simulink model "final"  (R2024a)
settings: Solver=VariableStepAuto  StartTime=0.0  StopTime=10.0  RelTol=1e-3
values from neighbouring files (symbols this model uses):
  A_air = 0.00588710854841    [run1.mat]    (also in run2.mat)
  Cs = 0.9    [run1.mat]    (also in run2.mat)
  h = 0.0127000254001    [run1.mat]    (also in run2.mat)
  m = 100    [run1.mat]    (also in run2.mat)
  T_f = 21    [run1.mat]    (also in run2.mat)
libraries: slctrl_linear x2, slpidlib x1
settings Model: Creator=veswaranandam  LastModifiedBy=veswaranandam

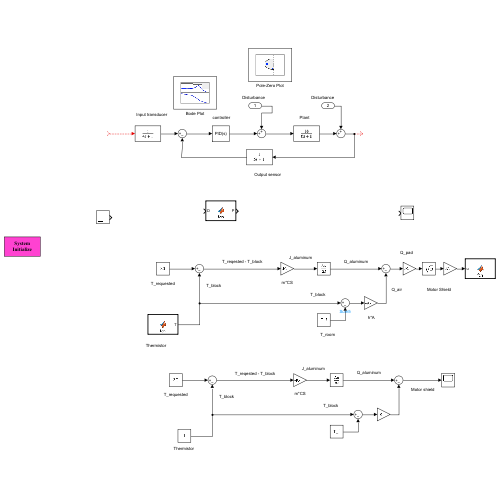
[thumbnail: Simulink's stored preview of the top-level diagram]
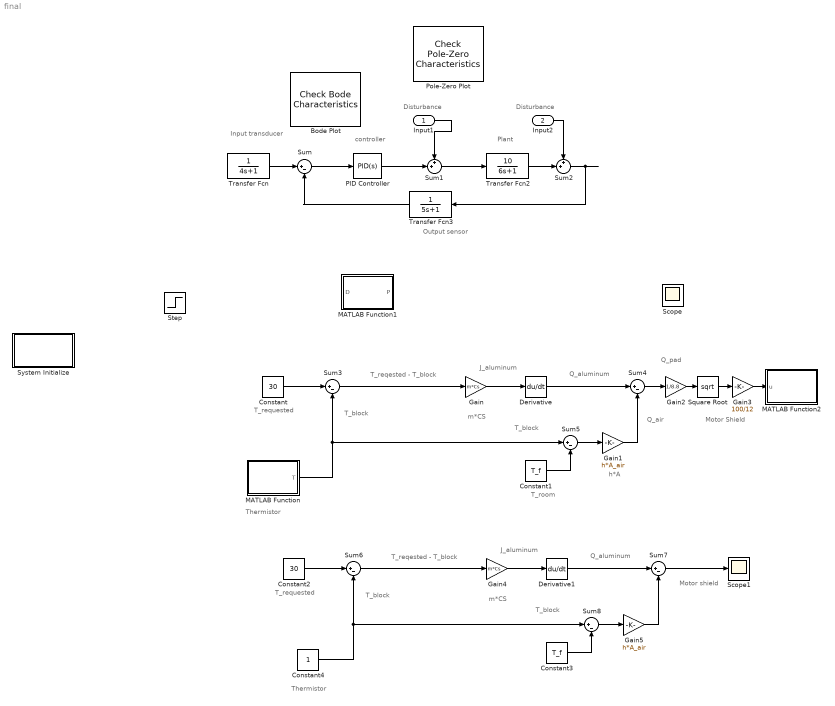
== system final ==
  note: Motor shield
  note: Thermistor
  note: T_block
  note: h*A
  note: T_room
  note: Q_pad
  note: Q_air
  note: Q_aluminum
  note: J_aluminum
  note: m*CS
  note: T_reqested - T_block
  note: T_block
  note: T_requested
  note: Motor Shield
  note: Thermistor
  note: Disturbance
  note: Disturbance
  note: controller
  note: Input transducer
  note: Plant
  note: Output sensor
  note: T_block
  note: J_aluminum
  note: Q_aluminum
  note: T_requested
  note: T_block
  note: m*CS
  note: T_reqested - T_block
  Input1 : Inport
  Input2 : Inport  Port=2
  Bode Plot : slctrl_linear/Check Bode  Characteristics  InstantiateOnLoad=on  SaveOperatingPoints=off  LinearizationIOs={'/Step', 1, 'in', 'off', '';'/Sum2', 1, 'out', 'off', ''}  LinearizeAt=SnapshotTimes  SnapshotTimes=[0]  TriggerType=rising  SampleTime=auto  RateConversionMethod=zoh  PreWarpFreq=10  UseExactDelayModel=off  UseFullBlockNameLabels=off  UseBusSignalLabels=off  enabled=on  stopWhenAssertionFail=off  export=off  ViewDlgPos=[385 83.4 509.6 389.6]  OpenViewOnLoad=off  LaunchViewOnOpen=on  FrequencyUnits=rad/s  MagnitudeUnits=dB  PhaseUnits=deg  TimeUnits=seconds  EnableUpperBound=off  UpperBoundFrequencies=[]  UpperBoundMagnitudes=[]  EnableLowerBound=off  LowerBoundFrequencies=[]  LowerBoundMagnitudes=[]
      settings: LibrarySourceBlock=slctrlblks/Linear Analysis Plots/Bode Plot  SaveToWorkspace=off  SaveName=sys
  Constant : Constant  Value=30
  Constant1 : Constant  Value=T_f
  Constant2 : Constant  Value=30
  Constant3 : Constant  Value=T_f
  Constant4 : Constant
  Derivative : Derivative
  Derivative1 : Derivative
  Gain : Gain  Gain=m*Cs
  Gain1 : Gain  Gain=h*A_air
  Gain2 : Gain  Gain=1/8.8
  Gain3 : Gain  Gain=100/12
  Gain4 : Gain  Gain=m*Cs
  Gain5 : Gain  Gain=h*A_air
  MATLAB Function : MATLAB Function  TreatAsAtomicUnit=on
  MATLAB Function1 : MATLAB Function  TreatAsAtomicUnit=on
  MATLAB Function2 : MATLAB Function  TreatAsAtomicUnit=on
  PID Controller : slpidlib/PID Controller  Controller=PID  Form=Parallel  TimeDomain=Continuous-time  UseExternalTs=off  SampleTime=-1  IntegratorMethod=Forward Euler  FilterMethod=Forward Euler  ControllerParametersSource=internal  P=0.91350417354806  I=0.0454811276391404  UseKiTs=off  D=-0.0153181987156712  UseExternalDerivativeSource=off  N=59.6352215103139  UseFilter=on  TunerSelectOption=Transfer Function Based (PID Tuner App)  InitialConditionSource=internal  InitialConditionForIntegrator=0  InitialConditionForFilter=0  DifferentiatorICPrevScaledInput=0  ExternalReset=none  TrackingMode=off  Kt=1  LimitOutput=off  SatLimitsSource=internal  UpperSaturationLimit=inf  LowerSaturationLimit=-inf  LinearizeAsGain=on  AntiWindupMode=none  Kb=1  LimitIntegrator=off  UpperIntegratorSaturationLimit=inf  LowerIntegratorSaturationLimit=-inf  POutMin=[]  POutMax=[]  IOutMin=[]  IOutMax=[]  DOutMin=[]  DOutMax=[]  NOutMin=[]  NOutMax=[]  SumOutMin=[]  SumOutMax=[]  SaturationOutMin=[]  SaturationOutMax=[]  PParamMin=[]  PParamMax=[]  IParamMin=[]  IParamMax=[]  DParamMin=[]  DParamMax=[]  NParamMin=[]  NParamMax=[]  KbParamMin=[]  KbParamMax=[]  KtParamMin=[]  KtParamMax=[]  KbOutMin=[]  KbOutMax=[]  KtOutMin=[]  KtOutMax=[]  IntegratorOutMin=[]  IntegratorOutMax=[]  FilterOutMin=[]  FilterOutMax=[]  SumI1OutMin=[]  SumI1OutMax=[]  SumI2OutMin=[]  SumI2OutMax=[]  SumI3OutMin=[]  SumI3OutMax=[]  SumI4OutMin=[]  SumI4OutMax=[]  SumDOutMin=[]  SumDOutMax=[]  DifferentiatorOutMin=[]  DifferentiatorOutMax=[]  FilterDiffOutCoefMin=[]  FilterDiffOutCoefMax=[]  ReciprocalOutMin=[]  ReciprocalOutMax=[]  SumDenOutMin=[]  SumDenOutMax=[]  SumNumOutMin=[]  SumNumOutMax=[]  DivideOutMin=[]  DivideOutMax=[]  UdiffTsProdOutMin=[]  UdiffTsProdOutMax=[]  NTsProdOutMin=[]  NTsProdOutMax=[]  UintegralTsProdOutMin=[]  UintegralTsProdOutMax=[]  UngainTsProdOutMin=[]  UngainTsProdOutMax=[]  ClampingZeroOutDataTypeStr=Inherit: Inherit via back propagation  ClampingZeroOutMin=[]  ClampingZeroOutMax=[]  FilterDenConstantOutDataTypeStr=Inherit: Inherit via back propagation  FilterDenConstantOutMin=[]  FilterDenConstantOutMax=[]  PCopyOutDataTypeStr=Inherit: Inherit via back propagation  PCopyOutMin=[]  PCopyOutMax=[]  NCopyOutDataTypeStr=Inherit: Inherit via back propagation  NCopyOutMin=[]  NCopyOutMax=[]  IntegratorContinuousStateAttributes=''  IntegratorStateMustResolveToSignalObject=off  IntegratorRTWStateStorageClass=Auto  FilterContinuousStateAttributes=''  FilterStateMustResolveToSignalObject=off  FilterRTWStateStorageClass=Auto  ParallelPVariant=InternalParameters  IdealPVariant=Disabled  IVariant=InternalParameters  DVariant=InternalParameters  IntegratorVariant=Continuous  SatVariant=Disabled  AWVariant=Passthrough  PCopyVariant=Disabled  TRVariant=Disabled  FdbkBlocksVariant=Forward  IdealPFdbkVariant=Disabled  SatFdbkVariant=Disabled  DerivativeFilterVariant=ContFilter  NVariant=InternalParameters  NCopyVariant=Disabled  FilterICVariant=InternalICsFilter  IntegratorICVariant=InternalICs  ExternalResetVariant=Disabled  TRSumVariant=Passthrough  SumFdbkVariant=Disabled  SumVariant=Sum_PID  TsampFilterVariant=InternalTs  TsampNgainVariant=Passthrough  TsampIntegralVariant=Disabled_SignalSpec  ExternalSaturationOutDataTypeStr=Inherit: Same as second input  DerivativeSourceVariant=ErrorSignal
  Pole-Zero Plot : slctrl_linear/Check Pole-Zero Characteristics  InstantiateOnLoad=on  SaveOperatingPoints=off  LinearizationIOs={'/Step', 1, 'in', 'off', '';'/Sum2', 1, 'out', 'off', ''}  LinearizeAt=SnapshotTimes  SnapshotTimes=[0]  TriggerType=rising  SampleTime=auto  RateConversionMethod=zoh  PreWarpFreq=10  UseExactDelayModel=off  UseFullBlockNameLabels=off  UseBusSignalLabels=off  enabled=on  stopWhenAssertionFail=off  export=off  ViewDlgPos=[887.4 121 509.6 389.6]  LaunchViewOnOpen=off  OpenViewOnLoad=on  FrequencyUnits=rad/s  MagnitudeUnits=dB  PhaseUnits=deg  TimeUnits=seconds  EnableSettlingTime=off  SettlingTime=[]  EnablePercentOvershoot=off  PercentOvershoot=[]  EnableDampingRatio=off  DampingRatio=[]  EnableNaturalFrequency=off  NaturalFrequencyBound=>=  NaturalFrequency=[]
      settings: LibrarySourceBlock=slctrlblks/Linear Analysis Plots/Pole-Zero Plot  SaveToWorkspace=off  SaveName=sys
  Scope : Scope
  Scope1 : Scope
  Square Root : Sqrt
  Step : Step  SampleTime=0
  Sum{,3..8} (7 alike) : Sum  Inputs=|+-
  Sum1 : Sum  Inputs=++|
  Sum2 : Sum  Inputs=++|
  System Initialize : Subsystem  mask(System Initialize){ShowInLibBrowser=0}
      mask prompts: ShowInLibBrowser "Simulink:masks:CustCodeMaskParam1_MP"
      settings: CopyFcn=cccopyfcn(gcb)  OpenFcn=ccopenfcn('System Initialize Function')
      mask Help: eval('feval(''rtwprivate'',''rtwhelpview'',''rtw_sys_initialize_block'')');
      mask Display: disp('System\nInitialize');
  Transfer Fcn : TransferFcn  Denominator=[4 1]
  Transfer Fcn2 : TransferFcn  Numerator=[10]  Denominator=[6 1]
  Transfer Fcn3 : TransferFcn  Denominator=[5 1]
  wires:
  Sum2/1 -> Transfer Fcn3/1
  Transfer Fcn2/1 -> Sum2/2
  Transfer Fcn3/1 -> Sum/2
  ? -> Transfer Fcn/1
  Transfer Fcn/1 -> Sum/1
  Sum/1 -> PID Controller/1
  Sum1/1 -> Transfer Fcn2/1
  PID Controller/1 -> Sum1/2
  Input1/1 -> Sum1/1
  Input2/1 -> Sum2/1
  Constant/1 -> Sum3/1
  Sum3/1 -> Gain/1
  Gain/1 -> Derivative/1
  Derivative/1 -> Sum4/1
  Constant1/1 -> Sum5/2
  Sum5/1 -> Gain1/1
  Gain1/1 -> Sum4/2
  MATLAB Function/1(T) -> Sum5/1, Sum3/2
  Sum4/1 -> Gain2/1
  Gain2/1 -> Square Root/1
  Square Root/1 -> Gain3/1
  Gain3/1 -> MATLAB Function2/1(u)
  Gain5/1 -> Sum7/2
  Gain4/1 -> Derivative1/1
  Sum8/1 -> Gain5/1
  Constant3/1 -> Sum8/2
  Constant2/1 -> Sum6/1
  Derivative1/1 -> Sum7/1
  Constant4/1 -> Sum8/1, Sum6/2
  Sum6/1 -> Gain4/1
  Sum7/1 -> Scope1/1

== system final/System Initialize ==

== matlab function final/MATLAB Function ==
  data: T output

function T = fcn()
    a = arduino("COM7","Uno");
    b = 3950;
    R25 = 10000;
    V_t = readVoltage(a,"A0");
    R_t = 10000/(5/V_t  - 1);
    T = 1/(log(R_t / R25)/b+1/298.15) - 273.15;

== matlab function final/MATLAB Function2 ==
  data: u input
function fcn(u)
    dcm.Speed(max(min(1,u),-1));

== matlab function final/MATLAB Function1 ==
  data: D input; P output
function P = fcn(D)
P = (12*D)^2 * 8.8;
